simulink model "untitled1"  (R2025a)
settings: Solver=VariableStepAuto  StartTime=0.0  StopTime=10.0  RelTol=1e-3

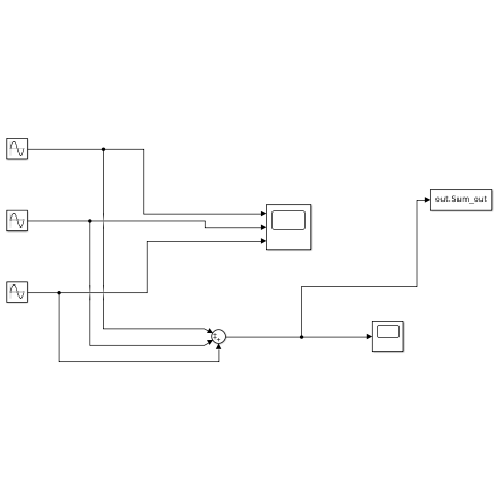
[thumbnail: Simulink's stored preview of the top-level diagram]
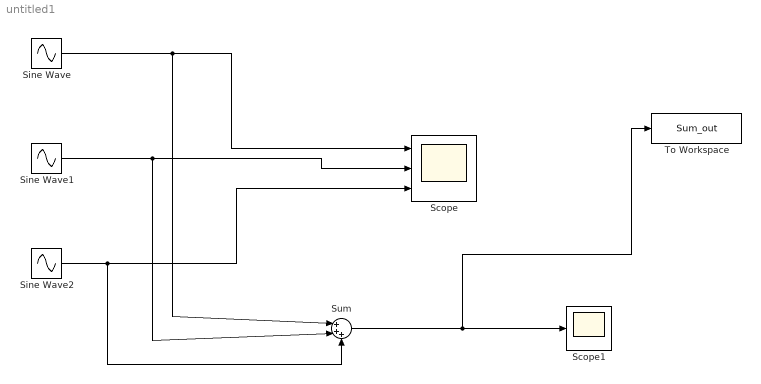
== system untitled1 ==
  Scope : Scope  NumInputPorts=3
      settings: ActiveDisplayYMinimum=-24.941746055094253  ActiveDisplayYMaximum=16.636817533133136
  Scope1 : Scope
      settings: ActiveDisplayYMinimum=-11.422195307356873  ActiveDisplayYMaximum=13.921347022140237
  Sine Wave : Sin  SampleTime=0
  Sine Wave1 : Sin  SampleTime=0
  Sine Wave2 : Sin  SampleTime=0
  Sum : Sum  Inputs=|+++
  To Workspace : ToWorkspace  VariableName=Sum_out  SaveFormat=Timeseries  SampleTime=-1
  wires:
  Sum/1 -> To Workspace/1, Scope1/1
  Sine Wave1/1 -> Sum/2, Scope/2
  Sine Wave2/1 -> Sum/3, Scope/3
  Sine Wave/1 -> Sum/1, Scope/1
